simulink model "lab_2_qpsk_sqrt_lpf_z"  (R2012b)
settings: Solver=ode45  StartTime=0.0  StopTime=0.0004  FixedStep=Td  RelTol=1e-3
values from neighbouring files (symbols this model uses):
  Fc = 2*pi*Rs    (= 2814867.01762)    [lab_2_parameters.m]
  Rb = Nvar*64000    (= 896000)    [lab_2_parameters.m]
  Rs = Rb/2    (= 448000)    [lab_2_parameters.m]
  Td = Ts/128    (= 1.74386160714e-08)    [lab_2_parameters.m]
  Ts = 1/Rs    (= 2.23214285714e-06)    [lab_2_parameters.m]
undefined symbols (not defined in the file or in its folder): dfilt, figposition, Fs, sided, Two
libraries: commsink2 x5, dspsrcs4 x4, dsparch4 x4, commfilt2 x4, commrandsrc2 x2, commdigbbndpm3 x2, dspsnks4 x2, commchan3 x1
settings Model: Creator=yuw  LastModifiedBy=yuw
settings OptimizationCC: InlineInvariantSignals=on  InitFltsAndDblsToZero=on
settings DebuggingCC: SaveWithParameterizedLinksMsg=none  SignalResolutionControl=TryResolveAllWithWarning  MultiTaskDSMMsg=warning  MultiTaskCondExecSysMsg=none  StrictBusMsg=None
settings RTWCC: IncludeERTFirstTime=on
settings GRTTargetCC: TargetFcnLib=ansi_tfl_tmw.mat  CombineOutputUpdateFcns=off  GRTInterface=on

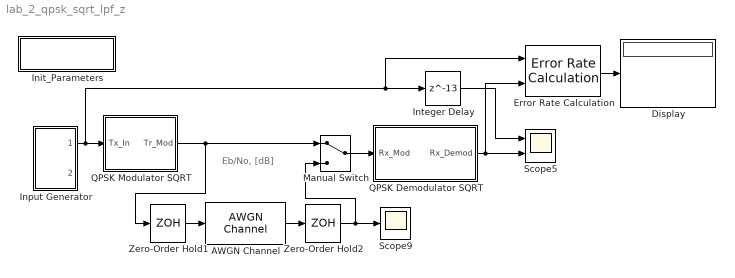
== system lab_2_qpsk_sqrt_lpf_z ==
  note: Eb/No, [dB]
  AWGN Channel : commchan3/AWGN Channel  InputProcessing=Columns as channels (frame based)  seed=56479  noiseMode="Signal to noise ratio  (Eb/No)"  EbNodB=5  EsNodB=20  SNRdB=10  bitsPerSym=1  Ps=1  Tsym=Ts  variance=1
  Display : Display
  Error Rate Calculation : commsink2/Error Rate Calculation  N=13  st_delay=0  cp_mode=Entire frame  subframe=[]  PMode=Port  WsName=ErrorVec  RsMode2=off  stop=off  numErr=100  maxBits=1e6
  Init_Parameters : Subsystem
      settings: OpenFcn=lab_2_parameters
      mask Display: disp('lab_2_parameters')
  Input Generator : Subsystem
  Integer Delay : Delay  DelayLength=13  InputProcessing=Inherited
  Manual Switch : ManualSwitch
  QPSK Demodulator SQRT : Subsystem
  QPSK Modulator SQRT : Subsystem
  Scope5 : Scope  NumInputPorts=2
      settings: TimeRange=5  YMin=-5~-5  YMax=5~5  SaveName=ScopeData5
  Scope9 : Scope
      settings: SaveName=ScopeData9
  Zero-Order Hold1 : ZeroOrderHold  SampleTime=Td
  Zero-Order Hold2 : ZeroOrderHold  SampleTime=Td
  wires:
  Error Rate Calculation/1 -> Display/1
  Zero-Order Hold2/1 -> Scope9/1, Manual Switch/2
  QPSK Modulator SQRT/1(Tr_Mod) -> Manual Switch/1, Zero-Order Hold1/1
  Manual Switch/1 -> QPSK Demodulator SQRT/1(Rx_Mod)
  Input Generator/1(Integer) -> QPSK Modulator SQRT/1(Tx_In), Integer Delay/1, Error Rate Calculation/1
  QPSK Demodulator SQRT/1(Rx_Demod) -> Error Rate Calculation/2, Scope5/2
  Integer Delay/1 -> Scope5/1
  AWGN Channel/1 -> Zero-Order Hold2/1
  Zero-Order Hold1/1 -> AWGN Channel/1

== system lab_2_qpsk_sqrt_lpf_z/Init_Parameters ==

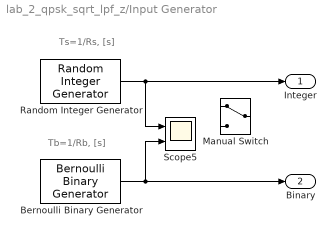
== system lab_2_qpsk_sqrt_lpf_z/Input Generator ==
  note: Ts=1/Rs, [s]
  note: Tb=1/Rb, [s]
  Bernoulli Binary Generator : commrandsrc2/Bernoulli Binary Generator  P=0.5  seed=12345  Ts=1/Rb  frameBased=off  sampPerFrame=1  orient=off  outDataType=double
  Manual Switch : ManualSwitch
  Random Integer Generator : commrandsrc2/Random Integer Generator  mul=4  seed=12345  Ts=1/Rs  frameBased=off  sampPerFrame=1  orient=off  outDataType=double
  Scope5 : Scope  NumInputPorts=2
      settings: TimeRange=5  YMin=-5~-5  YMax=5~5  SaveName=ScopeData11
  Integer : Outport
  Binary : Outport  Port=2
  wires:
  Random Integer Generator/1 -> Integer/1, Scope5/1
  Bernoulli Binary Generator/1 -> Scope5/2, Binary/1

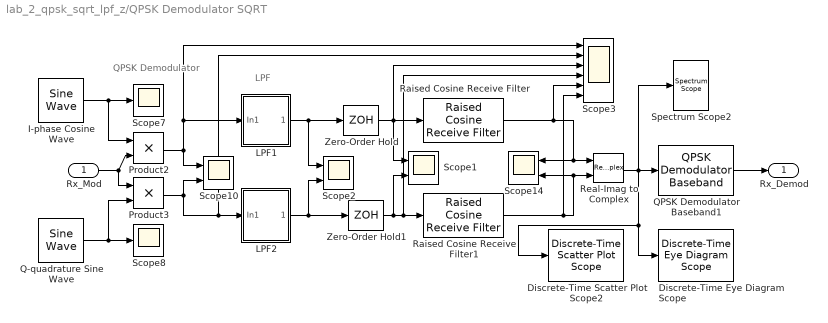
== system lab_2_qpsk_sqrt_lpf_z/QPSK Demodulator SQRT ==
  note: QPSK Demodulator
  note: LPF
  Rx_Mod : Inport
  Discrete-Time Eye Diagram Scope : commsink2/Discrete-Time Eye Diagram Scope  Tag=EyeDiagram  sampPerSymb=8  offsetEye=0  symbPerTrace=1  numTraces=40  numNewFrames=10  LineStyles=-  LineColors=b  dupPoints=on  fading=on  render=on  AxisGrid=on  yMin=-1.5  yMax=1.5  inphaseLabel=In-phase Amplitude  quadratureLabel=Quadrature Amplitude  openScopeAtSimStart=on  dispDiagram=In-phase and Quadrature  FrameNumber=off  FigPos=[360 54 560 644]  figTitle=Eye Diagram  block_type_=eye  numLinesMax=8
  Discrete-Time Scatter Plot Scope2 : commsink2/Discrete-Time Scatter Plot Scope  Tag=ScatterPlot  sampPerSymb=1  offsetEye=0  numTraces=40  numNewFrames=10  LineMarkers=.  LineColors=b  fading=on  render=on  AxisGrid=on  xMin=-1.5  xMax=1.5  yMin=-1.5  yMax=1.5  inphaseLabel=In-phase Amplitude  quadratureLabel=Quadrature Amplitude  openScopeAtSimStart=off  FrameNumber=off  FigPos=[360 138 560 560]  figTitle=Scatter Plot  numLinesMax=8  block_type_=scatter
  I-phase Cosine Wave : dspsrcs4/Sine Wave  Amplitude=sqrt(2)  Frequency=Fc  Phase=pi/2  SampleMode=Discrete  OutComplex=Real  CompMethod=Trigonometric fcn  TableSize=Speed  SampleTime=Td  SamplesPerFrame=1  ResetState=Restart at time zero  dataType=double  wordLen=16  udDataType=sfix(16)  fracBitsMode=Best precision  numFracBits=15  OutDataTypeStr=double  LastOutDataTypeStr=double
  LPF1 : Subsystem
  LPF2 : Subsystem
  Product2 : Product  SampleTime=Td  RndMeth=Zero
  Product3 : Product  SampleTime=Td  RndMeth=Zero
  Q-quadrature Sine Wave : dspsrcs4/Sine Wave  Amplitude=1  Frequency=Fc  Phase=pi  SampleMode=Discrete  OutComplex=Real  CompMethod=Trigonometric fcn  TableSize=Speed  SampleTime=Td  SamplesPerFrame=1  ResetState=Restart at time zero  dataType=double  wordLen=16  udDataType=sfix(16)  fracBitsMode=Best precision  numFracBits=15  OutDataTypeStr=double  LastOutDataTypeStr=double
  QPSK Demodulator Baseband1 : commdigbbndpm3/QPSK Demodulator Baseband  Ph=pi/4  Dec=Gray  OutType=Integer  DecType=Hard decision  VarSource=Dialog  Variance=1  outDtype1=Inherit via internal rule  outDtype2=Inherit via internal rule  derotateFactorWordLen=16
  Raised Cosine Receive Filter : commfilt2/Raised Cosine Receive Filter  filtType=Square root  N=8  D=6  R=0.2  sampMode=Mute  saveAsFlag=0  rateMode=Downsampling  downFactor=8  downOffset=0  framing=Maintain input frame size  checkGain=Normalized  filterGain=1  checkCoeff=off  variableName=rcRxFilt  launchFVT=off  roundingMode=Floor  overflowMode=off
  Raised Cosine Receive Filter1 : commfilt2/Raised Cosine Receive Filter  filtType=Square root  N=8  D=6  R=0.2  sampMode=Mute  saveAsFlag=0  rateMode=Downsampling  downFactor=8  downOffset=0  framing=Maintain input frame size  checkGain=Normalized  filterGain=1  checkCoeff=off  variableName=rcRxFilt1  launchFVT=off  roundingMode=Floor  overflowMode=off
  Real-Imag to Complex : RealImagToComplex
  Scope{1..2,10,14} (4 alike) : Scope  NumInputPorts=2
      Scope1 settings: YMin=-5~-5  YMax=5~5  SaveName=ScopeData12
      Scope10 settings: YMin=-5~-5  YMax=5~5  SaveName=ScopeData10
      Scope14 settings: TimeRange=5  YMin=-5~-5  YMax=5~5  SaveName=ScopeData4
      Scope2 settings: YMin=-5~-5  YMax=5~5  SaveName=ScopeData14
  Scope3 : Scope  NumInputPorts=6
      settings: YMin=-5~-5~-5~-5~-5~-5  YMax=5~5~5~5~5~5  SaveName=ScopeData15
  Scope7 : Scope
      settings: SaveName=ScopeData7
  Scope8 : Scope
      settings: SaveName=ScopeData8
  Spectrum Scope2 : dspsnks4/Spectrum Scope  ScopeProperties=on  Domain=Frequency  HorizSpan=1  UseBuffer=on  BufferSize=256  Overlap=0  TreatMby1Signals=M channels  inpFftLenInherit=off  FFTlength=128  numAvg=20  DisplayProperties=off  AxisGrid=on  Memory=off  FrameNumber=off  AxisLegend=off  AxisZoom=off  OpenScopeAtSimStart=on  OpenScopeImmediately=off  FigPos="figposition([49    12    39    27])"  AxisProperties=off  XUnits=Hertz  XRange=Two-sided ((-Fs/2...Fs/2])  XDisplay=0  InheritXIncr=on  XIncr=1.0  XLabel=Samples  XLimit=Auto  YUnits=dBW/Hertz  XMax=1  XMin=0  YLabel=Magnitude-squared, dB  LineProperties=off  LineColors=[1 0 0]  wintypeSpecScope=Hann  RsSpecScope=50  betaSpecScope=5  winsampSpecScope=Periodic  XAxisParamsVer=6.9  isFrameUpgraded=on
      settings: YMin=-10  YMax=10
  Zero-Order Hold : ZeroOrderHold  SampleTime=Ts/8
  Zero-Order Hold1 : ZeroOrderHold  SampleTime=1/Rs/8
  Rx_Demod : Outport
  wires:
  Product3/1 -> Scope10/2, LPF2/1(In1), Scope3/2
  Product2/1 -> Scope10/1, LPF1/1(In1), Scope3/1
  I-phase Cosine Wave/1 -> Scope7/1, Product2/1
  Q-quadrature Sine Wave/1 -> Scope8/1, Product3/2
  Real-Imag to Complex/1 -> QPSK Demodulator Baseband1/1, Discrete-Time Eye Diagram Scope/1, Discrete-Time Scatter Plot Scope2/1, Spectrum Scope2/1
  Rx_Mod/1 -> Product2/2, Product3/1
  QPSK Demodulator Baseband1/1 -> Rx_Demod/1
  Zero-Order Hold/1 -> Raised Cosine Receive Filter/1, Scope1/1, Scope3/3
  Zero-Order Hold1/1 -> Scope1/2, Raised Cosine Receive Filter1/1, Scope3/4
  LPF1/1(Out1) -> Zero-Order Hold/1, Scope2/1
  LPF2/1(Out1) -> Zero-Order Hold1/1, Scope2/2
  Raised Cosine Receive Filter1/1 -> Real-Imag to Complex/2, Scope14/2, Scope3/6
  Raised Cosine Receive Filter/1 -> Real-Imag to Complex/1, Scope14/1, Scope3/5

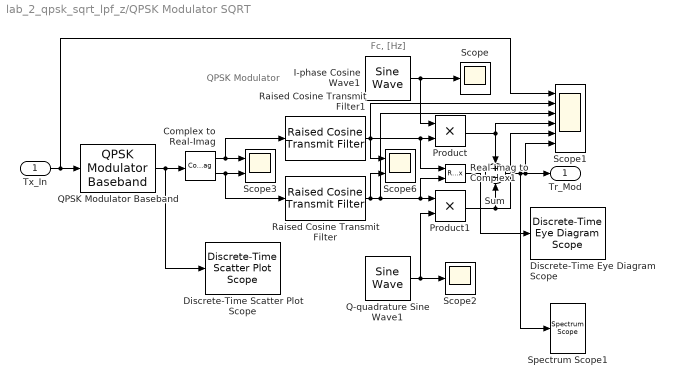
== system lab_2_qpsk_sqrt_lpf_z/QPSK Modulator SQRT ==
  note: QPSK Modulator
  note: Fc, [Hz]
  Tx_In : Inport
  Complex to Real-Imag : ComplexToRealImag
  Discrete-Time Eye Diagram Scope : commsink2/Discrete-Time Eye Diagram Scope  Tag=EyeDiagram  sampPerSymb=8  offsetEye=0  symbPerTrace=1  numTraces=40  numNewFrames=10  LineStyles=-  LineColors=b  dupPoints=on  fading=on  render=on  AxisGrid=on  yMin=-1.5  yMax=1.5  inphaseLabel=In-phase Amplitude  quadratureLabel=Quadrature Amplitude  openScopeAtSimStart=on  dispDiagram=In-phase and Quadrature  FrameNumber=off  FigPos=[360 54 560 644]  figTitle=Eye Diagram  block_type_=eye  numLinesMax=8
  Discrete-Time Scatter Plot Scope : commsink2/Discrete-Time Scatter Plot Scope  Tag=ScatterPlot  sampPerSymb=1  offsetEye=0  numTraces=40  numNewFrames=10  LineMarkers=.  LineColors=b  fading=on  render=on  AxisGrid=on  xMin=-1.5  xMax=1.5  yMin=-1.5  yMax=1.5  inphaseLabel=In-phase Amplitude  quadratureLabel=Quadrature Amplitude  openScopeAtSimStart=off  FrameNumber=off  FigPos=[360 138 560 560]  figTitle=Scatter Plot  numLinesMax=8  block_type_=scatter
  I-phase Cosine Wave1 : dspsrcs4/Sine Wave  Amplitude=sqrt(2)  Frequency=Fc  Phase=pi/2  SampleMode=Discrete  OutComplex=Real  CompMethod=Trigonometric fcn  TableSize=Speed  SampleTime=Td  SamplesPerFrame=1  ResetState=Restart at time zero  dataType=double  wordLen=16  udDataType=sfix(16)  fracBitsMode=Best precision  numFracBits=15  OutDataTypeStr=double  LastOutDataTypeStr=double
  Product : Product  RndMeth=Zero
  Product1 : Product  RndMeth=Zero
  Q-quadrature Sine Wave1 : dspsrcs4/Sine Wave  Amplitude=1  Frequency=Fc  Phase=0  SampleMode=Discrete  OutComplex=Real  CompMethod=Trigonometric fcn  TableSize=Speed  SampleTime=Td  SamplesPerFrame=1  ResetState=Restart at time zero  dataType=double  wordLen=16  udDataType=sfix(16)  fracBitsMode=Best precision  numFracBits=15  OutDataTypeStr=double  LastOutDataTypeStr=double
  QPSK Modulator Baseband : commdigbbndpm3/QPSK Modulator Baseband  InType=Integer  Enc=Gray  Ph=pi/4  outDtype=double  outWordLen=16  outUDDataType=sfix(16)  outFracLenMode=Best precision  outFracLen=15
  Raised Cosine Transmit Filter : commfilt2/Raised Cosine Transmit Filter  filtType=Square root  D=6  R=0.2  sampMode=Mute  saveAsFlag=0  N=8  framing=Maintain input frame size  checkGain=Normalized  filterGain=1  checkCoeff=off  variableName=rcTxFilt  launchFVT=off  roundingMode=Floor  overflowMode=off
  Raised Cosine Transmit Filter1 : commfilt2/Raised Cosine Transmit Filter  filtType=Square root  D=6  R=0.2  sampMode=Mute  saveAsFlag=0  N=8  framing=Maintain input frame size  checkGain=Normalized  filterGain=1  checkCoeff=off  variableName=rcTxFilt1  launchFVT=off  roundingMode=Floor  overflowMode=off
  Real-Imag to Complex1 : RealImagToComplex
  Scope : Scope
      settings: SaveName=ScopeData2
  Scope1 : Scope  NumInputPorts=6
      settings: TimeRange=5  YMin=-5~-5~-5~-5~-5~-5  YMax=5~5~5~5~5~5
  Scope2 : Scope
      settings: SaveName=ScopeData3
  Scope3 : Scope  NumInputPorts=2
      settings: YMin=-5~-5  YMax=5~5  SaveName=ScopeData13
  Scope6 : Scope  NumInputPorts=2
      settings: YMin=-5~-5  YMax=5~5  SaveName=ScopeData6
  Spectrum Scope1 : dspsnks4/Spectrum Scope  ScopeProperties=on  Domain=Frequency  HorizSpan=1  UseBuffer=on  BufferSize=256  Overlap=0  TreatMby1Signals=M channels  inpFftLenInherit=off  FFTlength=128  numAvg=20  DisplayProperties=off  AxisGrid=on  Memory=off  FrameNumber=off  AxisLegend=off  AxisZoom=off  OpenScopeAtSimStart=on  OpenScopeImmediately=off  FigPos="figposition([49    12    39    27])"  AxisProperties=off  XUnits=Hertz  XRange=Two-sided ((-Fs/2...Fs/2])  XDisplay=0  InheritXIncr=on  XIncr=1.0  XLabel=Samples  XLimit=Auto  YUnits=dBW/Hertz  XMax=1  XMin=0  YLabel=Magnitude-squared, dB  LineProperties=off  LineColors=[1 0 0]  wintypeSpecScope=Hann  RsSpecScope=50  betaSpecScope=5  winsampSpecScope=Periodic  XAxisParamsVer=6.9  isFrameUpgraded=on
      settings: YMin=-10  YMax=10
  Sum : Sum  Inputs=+-
  Tr_Mod : Outport
  wires:
  Product1/1 -> Sum/2, Scope1/5
  QPSK Modulator Baseband/1 -> Discrete-Time Scatter Plot Scope/1, Complex to Real-Imag/1
  Product/1 -> Sum/1, Scope1/4
  Sum/1 -> Tr_Mod/1, Scope1/6, Spectrum Scope1/1
  Tx_In/1 -> QPSK Modulator Baseband/1, Scope1/1
  Raised Cosine Transmit Filter/1 -> Scope6/2, Product1/1, Real-Imag to Complex1/2, Scope1/3
  I-phase Cosine Wave1/1 -> Product/1, Scope/1
  Q-quadrature Sine Wave1/1 -> Product1/2, Scope2/1
  Raised Cosine Transmit Filter1/1 -> Scope6/1, Product/2, Real-Imag to Complex1/1, Scope1/2
  Complex to Real-Imag/1 -> Raised Cosine Transmit Filter1/1, Scope3/1
  Complex to Real-Imag/2 -> Raised Cosine Transmit Filter/1, Scope3/2
  Real-Imag to Complex1/1 -> Discrete-Time Eye Diagram Scope/1

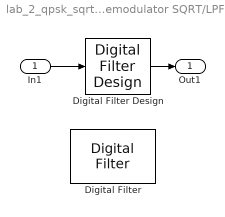
== system lab_2_qpsk_sqrt_lpf_z/QPSK Demodulator SQRT/LPF1 ==
  In1 : Inport
  Digital Filter Design : dsparch4/Digital Filter Design  mwdsp_browser_bugfix_var=off
  Digital Filter : dsparch4/Digital Filter  TypePopup=FIR (all zeros)  IIRFiltStruct=Direct form II transposed  AllPoleFiltStruct=Direct form  FIRFiltStruct=Direct form  CoeffSource=Specify via dialog  NumCoeffs=[1 2]  DenCoeffs=[1 0.1]  BiQuadCoeffs=[1 0.3 0.4 1 0.1 0.2]  LatticeCoeffs=[0.2 0.4]  denIgnore=on  FiltPerSampPopup=One filter per frame  IC=0  ICnum=0  ICden=0  roundingMode=Floor  overflowMode=off  ScaleValues=1  scaleValueFracLength=14  stageInFracLength=15  stageOutFracLength=15  FilterSource=Specify via dialog  dfiltObjectName=dfilt.dffir([1 2 1])
  Out1 : Outport
  wires:
  Digital Filter Design/1 -> Out1/1
  In1/1 -> Digital Filter Design/1

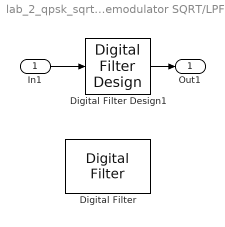
== system lab_2_qpsk_sqrt_lpf_z/QPSK Demodulator SQRT/LPF2 ==
  In1 : Inport
  Digital Filter Design1 : dsparch4/Digital Filter Design  mwdsp_browser_bugfix_var=off
  Digital Filter : dsparch4/Digital Filter  TypePopup=IIR (poles & zeros)  IIRFiltStruct=Direct form II transposed  AllPoleFiltStruct=Direct form  FIRFiltStruct=Direct form  CoeffSource=Specify via dialog  NumCoeffs=[1 2]  DenCoeffs=[1 0.1]  BiQuadCoeffs=[1 0.3 0.4 1 0.1 0.2]  LatticeCoeffs=[0.2 0.4]  denIgnore=on  FiltPerSampPopup=One filter per frame  IC=0  ICnum=0  ICden=0  roundingMode=Floor  overflowMode=off  ScaleValues=1  scaleValueFracLength=14  stageInFracLength=15  stageOutFracLength=15  FilterSource=Specify via dialog  dfiltObjectName=dfilt.dffir([1 2 1])
  Out1 : Outport
  wires:
  Digital Filter Design1/1 -> Out1/1
  In1/1 -> Digital Filter Design1/1
